simulink subsystem "RL_multi_switch_action"  (R2021a)
settings: Solver=VariableStepAuto  StartTime=0.0  StopTime=10.0  RelTol=1e-3
settings Model: Creator=tshintai  LastModifiedBy=tshintai

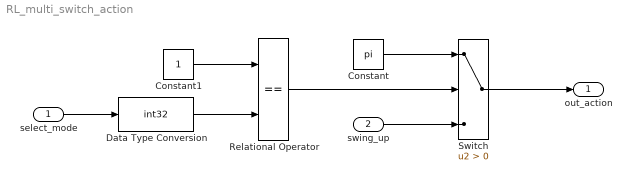
== system RL_multi_switch_action ==
  select_mode : Inport
  swing_up : Inport  Port=2
  Constant : Constant  Value=pi
  Constant1 : Constant  OutDataTypeStr=int32
  Data Type Conversion : DataTypeConversion  OutDataTypeStr=int32
  Relational Operator : RelationalOperator  Operator===  OutDataTypeStr=boolean  RndMeth=Simplest
  Switch : Switch  Criteria=u2 > Threshold
  out_action : Outport
  wires:
  select_mode/1 -> Data Type Conversion/1
  Data Type Conversion/1 -> Relational Operator/2
  Constant1/1 -> Relational Operator/1
  Relational Operator/1 -> Switch/2
  Constant/1 -> Switch/1
  swing_up/1 -> Switch/3
  Switch/1 -> out_action/1
